simulink model "engine_64"  (R2022b)
settings: Solver=ode45  StartTime=0.0  StopTime=timeFinal  MaxStep=timeStepMax  RelTol=1e-3
settings Model: Creator=jun  LastModifiedBy=jun

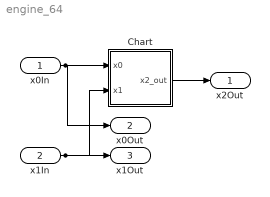
== system engine_64 ==
  x0In : Inport
  x1In : Inport  Port=2
  Chart : Stateflow chart  TreatAsAtomicUnit=on
  x2Out : Outport  SignalName=x2Out
  x0Out : Outport  Port=2  SignalName=x0Out
  x1Out : Outport  Port=3  SignalName=x1Out
  wires:
  x1In/1 -> x1Out/1, Chart/2(x1)
  Chart/1(x2_out) -> x2Out/1
  x0In/1 -> x0Out/1, Chart/1(x0)

== stateflow chart engine_64/Chart ==
  settings: updateMethod=CONTINUOUS  executeAtInitialization=1
  state loc1
    du:
    x2_dot = 172.1190893330591 * x0 + -18.178520839265644 * x1 + -0.5876147842465436 * x2 + 73.82076094915064 * 1;
    exit:
    x2_out = x2;
  state loc2
    du:
    x2_dot = 212.32859447747805 * x0 + -26.397573588389246 * x1 + -0.6081093746409181 * x2 + -30.45837836855404 * 1;
    exit:
    x2_out = x2;
  state loc3
    du:
    x2_dot = 344.54752773501156 * x0 + -35.88284070082604 * x1 + -0.9970388195562307 * x2 + -200.1049879468369 * 1;
    exit:
    x2_out = x2;
  state loc4
    du:
    x2_dot = 68.77841442397082 * x0 + -34.49189091176032 * x1 + 0.12328748344088325 * x2 + -1.3796756365879104 * 1;
    exit:
    x2_out = x2;
  state loc5
    du:
    x2_dot = 140.9675820907455 * x0 + -43.875858449678596 * x1 + -0.35477696051004415 * x2 + 521.9542303520906 * 1;
    exit:
    x2_out = x2;
  state loc6
    du:
    x2_dot = 302.8780197068835 * x0 + -44.80735860300237 * x1 + -0.9040556603935528 * x2 + 119.6620402089771 * 1;
    exit:
    x2_out = x2;
  state loc7
    du:
    x2_dot = 122.84651515781506 * x0 + -30.950644261836022 * x1 + -0.27788754543099614 * x2 + 165.80183448821774 * 1;
    exit:
    x2_out = x2;
  state loc8
    du:
    x2_dot = 167.10608158842408 * x0 + -108.5883262202008 * x1 + 0.009044623571327293 * x2 + 765.0984015639142 * 1;
    exit:
    x2_out = x2;
  state loc9
    du:
    x2_dot = 445.763959616979 * x0 + -48.47627467335269 * x1 + -2.0084227525216107 * x2 + 1229.5257992077045 * 1;
    exit:
    x2_out = x2;
  state loc10
    du:
    x2_dot = 498.3363297723553 * x0 + -608.1571396037069 * x1 + 2.2252382167093856 * x2 + -30.407856980192502 * 1;
    exit:
    x2_out = x2;
  state loc11
    du:
    x2_dot = 715.2746433139067 * x0 + -76.64137058300118 * x1 + -3.8995547737660843 * x2 + 4813.856810500421 * 1;
    exit:
    x2_out = x2;
  state loc12
    du:
    x2_dot = 101.74320415088494 * x0 + -1088.197236164022 * x1 + 10.09776041865507 * x2 + -54.40986180820271 * 1;
    exit:
    x2_out = x2;
  state loc13
    du:
    x2_dot = 0.9880803031927505 * x0 + 234.9676077852242 * x1 + -1.3449544898614079 * x2 + -2016.1925055525626 * 1;
    exit:
    x2_out = x2;
  state loc14
    du:
    x2_dot = 574.2410555812266 * x0 + -219.6862421234948 * x1 + -0.45181543339600694 * x2 + -8.78744968493992 * 1;
    exit:
    x2_out = x2;
  state loc15
    du:
    x2_dot = -113.62089642920859 * x0 + 1.4251893673222886 * x1 + 0.41547085892133473 * x2 + 0.07125946836611427 * 1;
    exit:
    x2_out = x2;
  state loc16
    du:
    x2_dot = -17.804841615106636 * x0 + -68.58762574035667 * x1 + 0.7167188324753084 * x2 + -3.4293812870178146 * 1;
    exit:
    x2_out = x2;
  state loc17
    du:
    x2_dot = 488.74438626957965 * x0 + 225.74711280684693 * x1 + -3.3008046366363715 * x2 + 11.287355640342154 * 1;
    exit:
    x2_out = x2;
  state loc18
    du:
    x2_dot = -468.38046258942035 * x0 + 2160.4248073159097 * x1 + -12.796021201925669 * x2 + 108.02124036578972 * 1;
    exit:
    x2_out = x2;
  state loc19
    du:
    x2_dot = 444.0255362071473 * x0 + -52.37346781168098 * x1 + -1.2930395931825203 * x2 + -108.66490645690529 * 1;
    exit:
    x2_out = x2;
  state loc20
    du:
    x2_dot = -869.7564517020274 * x0 + 109.0511700650369 * x1 + 2.8810707254181835 * x2 + -685.1892952940185 * 1;
    exit:
    x2_out = x2;
  state loc21
    du:
    x2_dot = 218.7833974995426 * x0 + -123.99564219310582 * x1 + -0.06817727388202854 * x2 + 761.9987134200146 * 1;
    exit:
    x2_out = x2;
  state loc22
    du:
    x2_dot = 788.4071927351927 * x0 + -119.82213911601772 * x1 + -2.006903759656254 * x2 + -5.991106955814446 * 1;
    exit:
    x2_out = x2;
  state loc23
    du:
    x2_dot = 423.7038947466738 * x0 + -43.16222518540387 * x1 + -1.3136762805154802 * x2 + -2.1581112592700946 * 1;
    exit:
    x2_out = x2;
  state loc24
    du:
    x2_dot = 994.6097170675433 * x0 + -203.68291006478168 * x1 + -2.1564190295835033 * x2 + -10.184145503239503 * 1;
    exit:
    x2_out = x2;
  state loc25
    du:
    x2_dot = 374.4538870917575 * x0 + -98.20167702486981 * x1 + -0.8107898899313994 * x2 + 419.8926588686644 * 1;
    exit:
    x2_out = x2;
  state loc26
    du:
    x2_dot = -244.70808961685935 * x0 + 19.943747525090956 * x1 + 0.7749081129909143 * x2 + 0.9971873762567732 * 1;
    exit:
    x2_out = x2;
  state loc27
    du:
    x2_dot = 411.98519906961934 * x0 + -620.8941581271833 * x1 + 2.744796134076182 * x2 + -31.04470790636005 * 1;
    exit:
    x2_out = x2;
  state loc28
    du:
    x2_dot = 808.0544999187772 * x0 + -453.71522052241687 * x1 + 0.16551686679935074 * x2 + -22.685761026118698 * 1;
    exit:
    x2_out = x2;
  state loc29
    du:
    x2_dot = 1233.9714475585872 * x0 + -154.78052698430878 * x1 + 1.7448402024567429 * x2 + -15821.406666081208 * 1;
    exit:
    x2_out = x2;
  state loc30
    du:
    x2_dot = 2676.133503156692 * x0 + -5868.971418919643 * x1 + 46.061341141875346 * x2 + -293.4485709459356 * 1;
    exit:
    x2_out = x2;
  state loc31
    du:
    x2_dot = 610.7207718994838 * x0 + -895.3235311192502 * x1 + 3.7777411657806397 * x2 + -44.76617655596021 * 1;
    exit:
    x2_out = x2;
  state loc32
    du:
    x2_dot = -3148.761851638217 * x0 + 10827.718842808368 * x1 + -93.44485779293609 * x2 + 541.3859421386076 * 1;
    exit:
    x2_out = x2;
  state loc33
    du:
    x2_dot = -12030.39472552258 * x0 + 25831.904809330747 * x1 + -205.25313427422952 * x2 + 1291.5952404673042 * 1;
    exit:
    x2_out = x2;
  state loc34
    du:
    x2_dot = 1263.8449377742227 * x0 + -2343.4654610634916 * x1 + 11.238228392457586 * x2 + -117.17327305316228 * 1;
    exit:
    x2_out = x2;
  state loc35
    du:
    x2_dot = 1182.9897670761286 * x0 + 2854.1817686159516 * x1 + -24.079857341380375 * x2 + 142.70908843089268 * 1;
    exit:
    x2_out = x2;
  state loc36
    du:
    x2_dot = 681.281153915759 * x0 + -678.712291850798 * x1 + 2.011639558995057 * x2 + -33.935614592536766 * 1;
    exit:
    x2_out = x2;
  state loc37
    du:
    x2_dot = 740.3742715734447 * x0 + 4.555906136101871 * x1 + -2.888094342106238 * x2 + 0.22779530681067664 * 1;
    exit:
    x2_out = x2;
  loc6 -> loc37 [order 20] : [ -1.0 * x0 + 0.0 * x1 + 0.013906389598449646 * x2 + -28.99226633725397 * 1 <= 0.000000 + 0]{x2 = 0.0 * x0 + 0.0 * x1 + 1.0 * x2 + 0.0; }
  loc31 -> loc2 [order 1] : [ 1.0 * x0 + 0.0 * x1 + -0.0004837518521937046 * x2 + -9.838665487841753 * 1 <= 0.000000 + 0]{x2 = 0.0 * x0 + 0.0 * x1 + 1.0 * x2 + 0.0; }
  loc30 -> loc1 [order 1] : [ 1.0 * x0 + 0.0 * x1 + 0.037800857937021634 * x2 + -86.5531921059513 * 1 <= 0.000000 + 0]{x2 = 0.0 * x0 + 0.0 * x1 + 1.0 * x2 + 0.0; }
  loc29 -> loc2 [order 1] : [ 1.0 * x0 + 0.0 * x1 + -0.003459682334038146 * x2 + -1.1898106761438398 * 1 <= 0.000000 + 0]{x2 = 0.0 * x0 + 0.0 * x1 + 1.0 * x2 + 0.0; }
  loc2 -> loc27 [order 16] : [ -1.0 * x0 + 0.0 * x1 + -0.04414154854203641 * x2 + 138.02065292561662 * 1 <= 0.000000 + 0]{x2 = 0.0 * x0 + 0.0 * x1 + 1.0 * x2 + 0.0; }
  loc29 -> loc5 [order 2] : [ 1.0 * x0 + 0.0 * x1 + -0.0006373591041330456 * x2 + -9.999681042268188 * 1 <= 0.000000 + 0]{x2 = 0.0 * x0 + 0.0 * x1 + 1.0 * x2 + 0.0; }
  loc27 -> loc5 [order 2] : [ 1.0 * x0 + 0.0 * x1 + -2.4418464604405856 * x2 + 7005.313200703071 * 1 <= 0.000000 + 0]{x2 = 0.0 * x0 + 0.0 * x1 + 1.0 * x2 + 0.0; }
  loc3 -> loc35 [order 15] : [ -1.0 * x0 + 0.0 * x1 + 0.013486455150813936 * x2 + -28.392022121626614 * 1 <= 0.000000 + 0]{x2 = 0.0 * x0 + 0.0 * x1 + 1.0 * x2 + 0.0; }
  loc1 -> loc32 [order 16] : [ -1.0 * x0 + 0.0 * x1 + 0.004088071137166638 * x2 + 0.2521195355914201 * 1 <= 0.000000 + 0]{x2 = 0.0 * x0 + 0.0 * x1 + 1.0 * x2 + 0.0; }
  loc25 -> loc6 [order 3] : [ -1.0 * x0 + 0.0 * x1 + 0.00966346036001345 * x2 + -17.678823102179155 * 1 <= 0.000000 + 0]{x2 = 0.0 * x0 + 0.0 * x1 + 1.0 * x2 + 0.0; }
  loc25 -> loc7 [order 4] : [ -1.0 * x0 + 0.0 * x1 + -0.0011937423705091499 * x2 + 15.265293647242267 * 1 <= 0.000000 + 0]{x2 = 0.0 * x0 + 0.0 * x1 + 1.0 * x2 + 0.0; }
  loc19 -> loc1 [order 1] : [ 1.0 * x0 + 0.0 * x1 + -4.5842158685289185e-05 * x2 + -8.34591726461707 * 1 <= 0.000000 + 0]{x2 = 0.0 * x0 + 0.0 * x1 + 1.0 * x2 + 0.0; }
  loc8 -> loc25 [order 13] : [ 1.0 * x0 + 0.0 * x1 + -0.008430233285089463 * x2 + 13.58360591452279 * 1 <= 0.000000 + 0]{x2 = 0.0 * x0 + 0.0 * x1 + 1.0 * x2 + 0.0; }
  loc28 -> loc11 [order 2] : [ -1.0 * x0 + 0.0 * x1 + 0.01341203766078607 * x2 + -28.164459590046405 * 1 <= 0.000000 + 0]{x2 = 0.0 * x0 + 0.0 * x1 + 1.0 * x2 + 0.0; }
  loc32 -> loc5 [order 1] : [ 1.0 * x0 + 0.0 * x1 + -0.02514010133359352 * x2 + 42.578630975660474 * 1 <= 0.000000 + 0]{x2 = 0.0 * x0 + 0.0 * x1 + 1.0 * x2 + 0.0; }
  loc20 -> loc5 [order 1] : [ -1.0 * x0 + 0.0 * x1 + 0.006990406418224249 * x2 + -5.009237016294506 * 1 <= 0.000000 + 0]{x2 = 0.0 * x0 + 0.0 * x1 + 1.0 * x2 + 0.0; }
  loc6 -> loc21 [order 14] : [ -1.0 * x0 + 0.0 * x1 + 0.002668645444580668 * x2 + 3.141070196132779 * 1 <= 0.000000 + 0]{x2 = 0.0 * x0 + 0.0 * x1 + 1.0 * x2 + 0.0; }
  loc6 -> loc31 [order 19] : [ -1.0 * x0 + 0.0 * x1 + 0.006683539436932168 * x2 + -8.706075096729139 * 1 <= 0.000000 + 0]{x2 = 0.0 * x0 + 0.0 * x1 + 1.0 * x2 + 0.0; }
  loc5 -> loc20 [order 15] : [ 1.0 * x0 + 0.0 * x1 + -0.0005830018611406415 * x2 + -7.805969915942764 * 1 <= 0.000000 + 0]{x2 = 0.0 * x0 + 0.0 * x1 + 1.0 * x2 + 0.0; }
  loc7 -> loc21 [order 8] : [ 1.0 * x0 + 0.0 * x1 + -0.011619069412716261 * x2 + 14.9354501584351 * 1 <= 0.000000 + 0]{x2 = 0.0 * x0 + 0.0 * x1 + 1.0 * x2 + 0.0; }
  loc5 -> loc18 [order 14] : [ 1.0 * x0 + 0.0 * x1 + -0.004338447137090646 * x2 + 1.1687838054601252 * 1 <= 0.000000 + 0]{x2 = 0.0 * x0 + 0.0 * x1 + 1.0 * x2 + 0.0; }
  loc1 -> loc14 [order 11] : [ -1.0 * x0 + 0.0 * x1 + 0.011364322618163452 * x2 + -21.491953472474837 * 1 <= 0.000000 + 0]{x2 = 0.0 * x0 + 0.0 * x1 + 1.0 * x2 + 0.0; }
  loc2 -> loc15 [order 11] : [ 1.0 * x0 + 0.0 * x1 + -0.005246642341844816 * x2 + 4.512806263509677 * 1 <= 0.000000 + 0]{x2 = 0.0 * x0 + 0.0 * x1 + 1.0 * x2 + 0.0; }
  loc2 -> loc23 [order 15] : [ -1.0 * x0 + 0.0 * x1 + -0.0066847022325267 * x2 + 31.03761365685755 * 1 <= 0.000000 + 0]{x2 = 0.0 * x0 + 0.0 * x1 + 1.0 * x2 + 0.0; }
  loc21 -> loc1 [order 1] : [ 1.0 * x0 + 0.0 * x1 + -0.03785322377042109 * x2 + 68.62399585559116 * 1 <= 0.000000 + 0]{x2 = 0.0 * x0 + 0.0 * x1 + 1.0 * x2 + 0.0; }
  loc17 -> loc6 [order 2] : [ 1.0 * x0 + 0.0 * x1 + 0.007876696914691554 * x2 + -35.52805351984629 * 1 <= 0.000000 + 0]{x2 = 0.0 * x0 + 0.0 * x1 + 1.0 * x2 + 0.0; }
  loc19 -> loc2 [order 2] : [ -1.0 * x0 + 2.1501424257403646e-14 * x1 + -0.49815175716791427 * x2 + 1497.204463041921 * 1 <= 0.000000 + 0]{x2 = 0.0 * x0 + 0.0 * x1 + 1.0 * x2 + 0.0; }
  loc25 -> loc8 [order 5] : [ 1.0 * x0 + 0.0 * x1 + -0.01386269505556377 * x2 + 19.586861582100134 * 1 <= 0.000000 + 0]{x2 = 0.0 * x0 + 0.0 * x1 + 1.0 * x2 + 0.0; }
  loc3 -> loc13 [order 10] : [ -1.0 * x0 + 0.0 * x1 + 0.00850238412940428 * x2 + -8.6891486981035 * 1 <= 0.000000 + 0]{x2 = 0.0 * x0 + 0.0 * x1 + 1.0 * x2 + 0.0; }
  loc16 -> loc6 [order 2] : [ -1.0 * x0 + 0.0 * x1 + 0.0010295685996749922 * x2 + 6.426480142622885 * 1 <= 0.000000 + 0]{x2 = 0.0 * x0 + 0.0 * x1 + 1.0 * x2 + 0.0; }
  loc9 -> loc1 [order 1] : [ 1.0 * x0 + 0.0 * x1 + 0.008495833391664445 * x2 + -25.608980012374634 * 1 <= 0.000000 + 0]{x2 = 0.0 * x0 + 0.0 * x1 + 1.0 * x2 + 0.0; }
  loc2 -> loc10 [order 10] : [ -1.0 * x0 + 0.0 * x1 + 0.013652563074296183 * x2 + -29.304627262579817 * 1 <= 0.000000 + 0]{x2 = 0.0 * x0 + 0.0 * x1 + 1.0 * x2 + 0.0; }
  loc13 -> loc21 [order 10] : [ -1.0 * x0 + 0.0 * x1 + 0.23556519772450607 * x2 + -669.100757040598 * 1 <= 0.000000 + 0]{x2 = 0.0 * x0 + 0.0 * x1 + 1.0 * x2 + 0.0; }
  loc8 -> loc21 [order 12] : [ 0.0 * x0 + 0.0 * x1 + -3.7019148417951926 * x2 + 7502.2921311782975 * 1 <= 0.000000 + 0]{x2 = 0.0 * x0 + 0.0 * x1 + 1.0 * x2 + 0.0; }
  loc6 -> loc19 [order 13] : [ -1.0 * x0 + 0.0 * x1 + 0.07262992925696107 * x2 + -136.64188709123505 * 1 <= 0.000000 + 0]{x2 = 0.0 * x0 + 0.0 * x1 + 1.0 * x2 + 0.0; }
  loc13 -> loc5 [order 4] : [ 1.0 * x0 + 0.0 * x1 + 0.0166038325905201 * x2 + -42.09105224715482 * 1 <= 0.000000 + 0]{x2 = 0.0 * x0 + 0.0 * x1 + 1.0 * x2 + 0.0; }
  loc13 -> loc6 [order 5] : [ -1.0 * x0 + 0.0 * x1 + 0.004000795211689418 * x2 + 0.3168817954571548 * 1 <= 0.000000 + 0]{x2 = 0.0 * x0 + 0.0 * x1 + 1.0 * x2 + 0.0; }
  loc1 -> loc13 [order 10] : [ -1.0 * x0 + 0.0 * x1 + 0.010412265577585919 * x2 + -15.559847318348758 * 1 <= 0.000000 + 0]{x2 = 0.0 * x0 + 0.0 * x1 + 1.0 * x2 + 0.0; }
  loc8 -> loc1 [order 1] : [ 1.0 * x0 + 0.0 * x1 + -0.0011841946054482308 * x2 + -6.817120131792731 * 1 <= 0.000000 + 0]{x2 = 0.0 * x0 + 0.0 * x1 + 1.0 * x2 + 0.0; }
  loc7 -> loc1 [order 1] : [ -1.0 * x0 + 0.0 * x1 + -0.000396194716564098 * x2 + 10.813484261025486 * 1 <= 0.000000 + 0]{x2 = 0.0 * x0 + 0.0 * x1 + 1.0 * x2 + 0.0; }
  loc7 -> loc2 [order 2] : [ 1.0 * x0 + 1.9355245087005833e-14 * x1 + -0.5842959775119011 * x2 + 1696.0577007802651 * 1 <= 0.000000 + 0]{x2 = 0.0 * x0 + 0.0 * x1 + 1.0 * x2 + 0.0; }
  loc10 -> loc2 [order 1] : [ -1.0 * x0 + 0.0 * x1 + -0.008129878521809913 * x2 + 35.3429710977038 * 1 <= 0.000000 + 0]{x2 = 0.0 * x0 + 0.0 * x1 + 1.0 * x2 + 0.0; }
  loc1 -> loc6 [order 5] : [ -1.0 * x0 + 1.920474508744948e-15 * x1 + 0.002396822510459467 * x2 + 3.886275756636265 * 1 <= 0.000000 + 0]{x2 = 0.0 * x0 + 0.0 * x1 + 1.0 * x2 + 0.0; }
  loc2 -> loc9 [order 9] : [ 1.0 * x0 + 0.0 * x1 + -0.0004847832930982423 * x2 + -8.002702057926387 * 1 <= 0.000000 + 0]{x2 = 0.0 * x0 + 0.0 * x1 + 1.0 * x2 + 0.0; }
  loc6 -> loc2 [order 2] : [ -1.0 * x0 + -2.2612069380927382e-14 * x1 + 0.0008976844746347977 * x2 + 7.987968808200821 * 1 <= 0.000000 + 0]{x2 = 0.0 * x0 + 0.0 * x1 + 1.0 * x2 + 0.0; }
  loc5 -> loc9 [order 9] : [ 1.0 * x0 + 0.0 * x1 + -0.02627481784478791 * x2 + 44.3802704365903 * 1 <= 0.000000 + 0]{x2 = 0.0 * x0 + 0.0 * x1 + 1.0 * x2 + 0.0; }
  loc3 -> loc9 [order 9] : [ 1.0 * x0 + 0.0 * x1 + 0.02989985141165207 * x2 + -68.67750395221753 * 1 <= 0.000000 + 0]{x2 = 0.0 * x0 + 0.0 * x1 + 1.0 * x2 + 0.0; }
  loc8 -> loc2 [order 2] : [ 1.0 * x0 + 0.0 * x1 + -0.004360712734463186 * x2 + 0.924986077398196 * 1 <= 0.000000 + 0]{x2 = 0.0 * x0 + 0.0 * x1 + 1.0 * x2 + 0.0; }
  loc5 -> loc8 [order 8] : [ -1.0 * x0 + 0.0 * x1 + -0.3165002257184714 * x2 + 802.3004669529307 * 1 <= 0.000000 + 0]{x2 = 0.0 * x0 + 0.0 * x1 + 1.0 * x2 + 0.0; }
  loc16 -> loc13 [order 3] : [ -1.0 * x0 + 0.0 * x1 + 0.003592581833683608 * x2 + 0.8675894511976858 * 1 <= 0.000000 + 0]{x2 = 0.0 * x0 + 0.0 * x1 + 1.0 * x2 + 0.0; }
  loc6 -> loc9 [order 8] : [ 1.0 * x0 + 0.0 * x1 + 0.012514221631630334 * x2 + -33.66438324655323 * 1 <= 0.000000 + 0]{x2 = 0.0 * x0 + 0.0 * x1 + 1.0 * x2 + 0.0; }
  loc1 -> loc5 [order 4] : [ -1.0 * x0 + -2.6266718131235672e-14 * x1 + 0.0008845513854542847 * x2 + 7.954499085333239 * 1 <= 0.000000 + 0]{x2 = 0.0 * x0 + 0.0 * x1 + 1.0 * x2 + 0.0; }
  loc5 -> loc2 [order 2] : [ 1.0 * x0 + 5.0921810950735284e-14 * x1 + -0.02049676115225059 * x2 + 41.34643404703749 * 1 <= 0.000000 + 0]{x2 = 0.0 * x0 + 0.0 * x1 + 1.0 * x2 + 0.0; }
  loc2 -> loc5 [order 5] : [ -1.0 * x0 + -6.107671307757277e-14 * x1 + -0.1353375334038646 * x2 + 411.09517067157344 * 1 <= 0.000000 + 0]{x2 = 0.0 * x0 + 0.0 * x1 + 1.0 * x2 + 0.0; }
  loc7 -> loc3 [order 3] : [ 1.0 * x0 + 0.0 * x1 + -0.0010294929919228354 * x2 + -7.2614381063231885 * 1 <= 0.000000 + 0]{x2 = 0.0 * x0 + 0.0 * x1 + 1.0 * x2 + 0.0; }
  loc2 -> loc4 [order 4] : [ 1.0 * x0 + 0.0 * x1 + -0.00016505883538827908 * x2 + -8.64187436094922 * 1 <= 0.000000 + 0]{x2 = 0.0 * x0 + 0.0 * x1 + 1.0 * x2 + 0.0; }
  loc5 -> loc3 [order 3] : [ 1.0 * x0 + 0.0 * x1 + -0.0008682788409220731 * x2 + -7.647835038707683 * 1 <= 0.000000 + 0]{x2 = 0.0 * x0 + 0.0 * x1 + 1.0 * x2 + 0.0; }
  loc6 -> loc3 [order 3] : [ 1.0 * x0 + 0.0 * x1 + 0.019351697137556877 * x2 + -58.86799090745678 * 1 <= 0.000000 + 0]{x2 = 0.0 * x0 + 0.0 * x1 + 1.0 * x2 + 0.0; }
  loc6 -> loc8 [order 7] : [ -1.0 * x0 + 0.0 * x1 + 0.01900167156417144 * x2 + -29.88892120409554 * 1 <= 0.000000 + 0]{x2 = 0.0 * x0 + 0.0 * x1 + 1.0 * x2 + 0.0; }
  loc7 -> loc8 [order 7] : [ 1.0 * x0 + 0.0 * x1 + -0.04280097395098223 * x2 + 93.25578195856991 * 1 <= 0.000000 + 0]{x2 = 0.0 * x0 + 0.0 * x1 + 1.0 * x2 + 0.0; }
  loc18 -> loc19 [order 1] : [ -1.0 * x0 + 0.0 * x1 + -0.0007374404508494473 * x2 + 13.516688409477354 * 1 <= 0.000000 + 0]{x2 = 0.0 * x0 + 0.0 * x1 + 1.0 * x2 + 0.0; }
  loc3 -> loc4 [order 4] : [ 1.0 * x0 + 0.0 * x1 + 0.001053045477463381 * x2 + -11.078191168027793 * 1 <= 0.000000 + 0]{x2 = 0.0 * x0 + 0.0 * x1 + 1.0 * x2 + 0.0; }
  loc5 -> loc4 [order 4] : [ 1.0 * x0 + 0.0 * x1 + -0.0002327516748476991 * x2 + -8.506449954332243 * 1 <= 0.000000 + 0]{x2 = 0.0 * x0 + 0.0 * x1 + 1.0 * x2 + 0.0; }
  loc2 -> loc3 [order 3] : [ 1.0 * x0 + 2.587408275651915e-14 * x1 + -0.00033074273625259185 * x2 + -9.139048550165036 * 1 <= 0.000000 + 0]{x2 = 0.0 * x0 + 0.0 * x1 + 1.0 * x2 + 0.0; }
  loc9 -> loc8 [order 6] : [ 1.0 * x0 + 0.0 * x1 + 0.0002770668648333768 * x2 + -8.995542602209866 * 1 <= 0.000000 + 0]{x2 = 0.0 * x0 + 0.0 * x1 + 1.0 * x2 + 0.0; }
  (junction 38) -> loc1 : [-1.0 * x0 + 9.775494234578627e-15 * x1 + 0.0121850121227071 * x2 + -21.54718632368986 * 1 <= 0.000000 + 0]{x2 = 0.0 * x0 + 0.0 * x1 + 1.0 * x2 + 0.0; }
  (default) -> loc1 : {x2 = a2; }
  (junction 77) -> loc2 : {x2 = x2; }
  (junction 60) -> loc2 : [-1.0 * x0 + 1.80572554083749e-15 * x1 + -0.0897209572126218 * x2 + 275.1294182888892 * 1 <= 0.000000 + 0]{x2 = 0.0 * x0 + 0.0 * x1 + 1.0 * x2 + 0.0; }
  (junction 97) -> loc3 : {x2 = x2; }
  (junction 82) -> loc3 : [1.0 * x0 + 0.0 * x1 + 0.005128621719638715 * x2 + -22.854840694945942 * 1 <= 0.000000 + 0]{x2 = 0.0 * x0 + 0.0 * x1 + 1.0 * x2 + 0.0; }
  (junction 101) -> loc4 : {x2 = x2; }
  (junction 125) -> loc5 : {x2 = x2; }
  (junction 108) -> loc5 : [1.0 * x0 + -8.853049182917268e-14 * x1 + -0.05600468311549547 * x2 + 125.14797413040408 * 1 <= 0.000000 + 0]{x2 = 0.0 * x0 + 0.0 * x1 + 1.0 * x2 + 0.0; }
  (junction 150) -> loc6 : {x2 = x2; }
  (junction 132) -> loc6 : [-1.0 * x0 + 8.119871136734383e-15 * x1 + 0.0043214885731190705 * x2 + -0.7481009740519966 * 1 <= 0.000000 + 0]{x2 = 0.0 * x0 + 0.0 * x1 + 1.0 * x2 + 0.0; }
  (junction 163) -> loc7 : {x2 = x2; }
  (junction 158) -> loc7 : [-1.0 * x0 + 2.3628053529496597e-15 * x1 + -0.0012646308978708435 * x2 + 14.00654036505749 * 1 <= 0.000000 + 0]{x2 = 0.0 * x0 + 0.0 * x1 + 1.0 * x2 + 0.0; }
  (junction 184) -> loc8 : {x2 = x2; }
  (junction 172) -> loc8 : [1.0 * x0 + 0.0 * x1 + -0.15658104490158298 * x2 + 373.13046083466145 * 1 <= 0.000000 + 0]{x2 = 0.0 * x0 + 0.0 * x1 + 1.0 * x2 + 0.0; }
  (junction 193) -> loc9 : {x2 = x2; }
  (junction 197) -> loc10 : {x2 = x2; }
  (junction 203) -> loc11 : {x2 = x2; }
  (junction 208) -> loc12 : {x2 = x2; }
  (junction 223) -> loc13 : {x2 = x2; }
  (junction 219) -> loc13 : [-1.0 * x0 + 0.0 * x1 + 0.003075190697417944 * x2 + 2.1890451934694903 * 1 <= 0.000000 + 0]{x2 = 0.0 * x0 + 0.0 * x1 + 1.0 * x2 + 0.0; }
  (junction 228) -> loc14 : {x2 = x2; }
  (junction 233) -> loc15 : {x2 = x2; }
  (junction 239) -> loc16 : {x2 = x2; }
  (junction 245) -> loc17 : {x2 = x2; }
  (junction 249) -> loc18 : {x2 = x2; }
  (junction 256) -> loc19 : {x2 = x2; }
  (junction 261) -> loc20 : {x2 = x2; }
  (junction 268) -> loc21 : {x2 = x2; }
  (junction 273) -> loc22 : {x2 = x2; }
  (junction 279) -> loc23 : {x2 = x2; }
  (junction 284) -> loc24 : {x2 = x2; }
  (junction 292) -> loc25 : {x2 = x2; }
  (junction 297) -> loc26 : {x2 = x2; }
  (junction 302) -> loc27 : {x2 = x2; }
  (junction 308) -> loc28 : {x2 = x2; }
  (junction 313) -> loc29 : {x2 = x2; }
  (junction 317) -> loc30 : {x2 = x2; }
  (junction 321) -> loc31 : {x2 = x2; }
  (junction 325) -> loc32 : {x2 = x2; }
  (junction 329) -> loc33 : {x2 = x2; }
  (junction 333) -> loc34 : {x2 = x2; }
  (junction 337) -> loc35 : {x2 = x2; }
  (junction 341) -> loc36 : {x2 = x2; }
  (junction 345) -> loc37 : {x2 = x2; }
  loc1 -> (junction 56) [order 17]
  (junction 56) -> loc1 : {x2 = x2; }
  loc1 -> (junction 38) [order 1]
  loc2 -> (junction 77) [order 17]
  loc2 -> (junction 60) [order 2]
  loc3 -> (junction 97) [order 16]
  loc3 -> (junction 82) [order 3]
  loc4 -> (junction 101) [order 2]
  loc5 -> (junction 125) [order 20]
  loc5 -> (junction 108) [order 5]
  loc6 -> (junction 150) [order 21]
  loc6 -> (junction 132) [order 5]
  loc7 -> (junction 163) [order 9]
  loc7 -> (junction 158) [order 6]
  loc8 -> (junction 184) [order 17]
  loc8 -> (junction 172) [order 7]
  loc9 -> (junction 193) [order 7]
  loc10 -> (junction 197) [order 2]
  loc11 -> (junction 203) [order 4]
  loc12 -> (junction 208) [order 3]
  loc13 -> (junction 223) [order 11]
  loc13 -> (junction 219) [order 9]
  loc14 -> (junction 228) [order 3]
  loc15 -> (junction 233) [order 3]
  loc16 -> (junction 239) [order 4]
  loc17 -> (junction 245) [order 4]
  loc18 -> (junction 249) [order 2]
  loc19 -> (junction 256) [order 5]
  loc20 -> (junction 261) [order 3]
  loc21 -> (junction 268) [order 5]
  loc22 -> (junction 273) [order 3]
  loc23 -> (junction 279) [order 4]
  loc24 -> (junction 284) [order 3]
  loc25 -> (junction 292) [order 6]
  loc26 -> (junction 297) [order 3]
  loc27 -> (junction 302) [order 3]
  loc28 -> (junction 308) [order 4]
  loc29 -> (junction 313) [order 3]
  loc30 -> (junction 317) [order 2]
  loc31 -> (junction 321) [order 2]
  loc32 -> (junction 325) [order 2]
  loc33 -> (junction 329) [order 2]
  loc34 -> (junction 333) [order 2]
  loc35 -> (junction 337) [order 2]
  loc36 -> (junction 341) [order 2]
  loc37 -> (junction 345) [order 2]
  loc6 -> loc11 [order 9] : [ -1.0 * x0 + 0.0 * x1 + 0.003061995106964173 * x2 + 2.727600433090311 * 1 <= 0.000000 + 0]{x2 = 0.0 * x0 + 0.0 * x1 + 1.0 * x2 + 0.0; }
  loc6 -> loc24 [order 15] : [ 1.0 * x0 + 0.0 * x1 + 0.0003851795086086663 * x2 + -9.224248852383578 * 1 <= 0.000000 + 0]{x2 = 0.0 * x0 + 0.0 * x1 + 1.0 * x2 + 0.0; }
  loc17 -> loc36 [order 3] : [ -1.0 * x0 + 0.0 * x1 + 0.0078073515693894355 * x2 + -12.275851653089429 * 1 <= 0.000000 + 0]{x2 = 0.0 * x0 + 0.0 * x1 + 1.0 * x2 + 0.0; }
  loc8 -> loc13 [order 8] : [ 1.0 * x0 + 0.0 * x1 + -0.41473185044808303 * x2 + 833.6030054148777 * 1 <= 0.000000 + 0]{x2 = 0.0 * x0 + 0.0 * x1 + 1.0 * x2 + 0.0; }
  loc8 -> loc28 [order 14] : [ 1.0 * x0 + 0.0 * x1 + -0.0008137390729368074 * x2 + -9.884470033609494 * 1 <= 0.000000 + 0]{x2 = 0.0 * x0 + 0.0 * x1 + 1.0 * x2 + 0.0; }
  loc28 -> loc29 [order 3] : [ -1.0 * x0 + 0.0 * x1 + 0.01198396513255497 * x2 + -23.96741959343518 * 1 <= 0.000000 + 0]{x2 = 0.0 * x0 + 0.0 * x1 + 1.0 * x2 + 0.0; }
  loc28 -> loc5 [order 1] : [ -1.0 * x0 + 0.0 * x1 + 0.014221919409240433 * x2 + -30.244302553187396 * 1 <= 0.000000 + 0]{x2 = 0.0 * x0 + 0.0 * x1 + 1.0 * x2 + 0.0; }
  loc8 -> loc7 [order 6] : [ 1.0 * x0 + 0.0 * x1 + -0.0005897625708588623 * x2 + -9.820014728923372 * 1 <= 0.000000 + 0]{x2 = 0.0 * x0 + 0.0 * x1 + 1.0 * x2 + 0.0; }
  loc1 -> loc7 [order 6] : [ -1.0 * x0 + 0.0 * x1 + 0.0006725296527658178 * x2 + 8.44586008456916 * 1 <= 0.000000 + 0]{x2 = 0.0 * x0 + 0.0 * x1 + 1.0 * x2 + 0.0; }
  loc1 -> loc16 [order 12] : [ -1.0 * x0 + 0.0 * x1 + 0.006938432653440454 * x2 + -5.844851815434497 * 1 <= 0.000000 + 0]{x2 = 0.0 * x0 + 0.0 * x1 + 1.0 * x2 + 0.0; }
  loc17 -> loc1 [order 1] : [ -1.0 * x0 + 0.0 * x1 + 0.009958076561476438 * x2 + -18.52621545079124 * 1 <= 0.000000 + 0]{x2 = 0.0 * x0 + 0.0 * x1 + 1.0 * x2 + 0.0; }
  loc26 -> loc13 [order 2] : [ -1.0 * x0 + 0.0 * x1 + 0.005272701492981822 * x2 + -2.24677477710992 * 1 <= 0.000000 + 0]{x2 = 0.0 * x0 + 0.0 * x1 + 1.0 * x2 + 0.0; }
  loc6 -> loc1 [order 1] : [ -1.0 * x0 + 5.2775269187444e-15 * x1 + 0.0018543047641648885 * x2 + 5.461340165715162 * 1 <= 0.000000 + 0]{x2 = 0.0 * x0 + 0.0 * x1 + 1.0 * x2 + 0.0; }
  loc3 -> loc5 [order 5] : [ -1.0 * x0 + 5.419359270896986e-16 * x1 + 6.766680895445332e-06 * x2 + 9.776387147649764 * 1 <= 0.000000 + 0]{x2 = 0.0 * x0 + 0.0 * x1 + 1.0 * x2 + 0.0; }
  loc3 -> loc24 [order 11] : [ -1.0 * x0 + 0.0 * x1 + 0.00020032908282740537 * x2 + 8.055033640322778 * 1 <= 0.000000 + 0]{x2 = 0.0 * x0 + 0.0 * x1 + 1.0 * x2 + 0.0; }
  loc15 -> loc6 [order 2] : [ -1.0 * x0 + 0.0 * x1 + 0.01247769896472895 * x2 + -24.822269825283854 * 1 <= 0.000000 + 0]{x2 = 0.0 * x0 + 0.0 * x1 + 1.0 * x2 + 0.0; }
  loc13 -> loc3 [order 3] : [ 1.0 * x0 + 0.0 * x1 + 0.0004328989487972267 * x2 + -9.385572117121479 * 1 <= 0.000000 + 0]{x2 = 0.0 * x0 + 0.0 * x1 + 1.0 * x2 + 0.0; }
  loc5 -> loc12 [order 10] : [ 1.0 * x0 + 0.0 * x1 + -0.15172077374063186 * x2 + 305.2791759295456 * 1 <= 0.000000 + 0]{x2 = 0.0 * x0 + 0.0 * x1 + 1.0 * x2 + 0.0; }
  loc5 -> loc22 [order 16] : [ 1.0 * x0 + 0.0 * x1 + -0.0007949504326678048 * x2 + -7.575308489923387 * 1 <= 0.000000 + 0]{x2 = 0.0 * x0 + 0.0 * x1 + 1.0 * x2 + 0.0; }
  loc9 -> loc7 [order 5] : [ 1.0 * x0 + 0.0 * x1 + 0.0011003152683534661 * x2 + -10.652779963478437 * 1 <= 0.000000 + 0]{x2 = 0.0 * x0 + 0.0 * x1 + 1.0 * x2 + 0.0; }
  loc9 -> loc3 [order 2] : [ 1.0 * x0 + 0.0 * x1 + 0.000505959707536987 * x2 + -9.50844114152303 * 1 <= 0.000000 + 0]{x2 = 0.0 * x0 + 0.0 * x1 + 1.0 * x2 + 0.0; }
  loc27 -> loc2 [order 1] : [ 1.0 * x0 + 0.0 * x1 + -0.003973753558748778 * x2 + 0.22232396459730006 * 1 <= 0.000000 + 0]{x2 = 0.0 * x0 + 0.0 * x1 + 1.0 * x2 + 0.0; }
  loc20 -> loc6 [order 2] : [ -1.0 * x0 + 0.0 * x1 + 0.003266853868709181 * x2 + 1.8536354335135146 * 1 <= 0.000000 + 0]{x2 = 0.0 * x0 + 0.0 * x1 + 1.0 * x2 + 0.0; }
  loc16 -> loc1 [order 1] : [ -1.0 * x0 + 0.0 * x1 + 0.07875374856763548 * x2 + -155.01450193772223 * 1 <= 0.000000 + 0]{x2 = 0.0 * x0 + 0.0 * x1 + 1.0 * x2 + 0.0; }
  loc2 -> loc6 [order 6] : [ -1.0 * x0 + 0.0 * x1 + -0.0007583640662728963 * x2 + 11.824030994291618 * 1 <= 0.000000 + 0]{x2 = 0.0 * x0 + 0.0 * x1 + 1.0 * x2 + 0.0; }
  loc2 -> loc17 [order 12] : [ 1.0 * x0 + 0.0 * x1 + -0.005947958362593438 * x2 + 6.6352236195673795 * 1 <= 0.000000 + 0]{x2 = 0.0 * x0 + 0.0 * x1 + 1.0 * x2 + 0.0; }
  loc11 -> loc2 [order 1] : [ -1.0 * x0 + 1.038173439278966e-15 * x1 + -0.01497800762556828 * x2 + 55.39052847424546 * 1 <= 0.000000 + 0]{x2 = 0.0 * x0 + 0.0 * x1 + 1.0 * x2 + 0.0; }
  loc5 -> loc1 [order 1] : [ 1.0 * x0 + 0.0 * x1 + -0.0037659877969931253 * x2 + -3.4088490147256745 * 1 <= 0.000000 + 0]{x2 = 0.0 * x0 + 0.0 * x1 + 1.0 * x2 + 0.0; }
  loc25 -> loc5 [order 2] : [ 1.0 * x0 + 0.0 * x1 + -0.0019058969268201038 * x2 + -6.262145480107898 * 1 <= 0.000000 + 0]{x2 = 0.0 * x0 + 0.0 * x1 + 1.0 * x2 + 0.0; }
  loc22 -> loc1 [order 1] : [ 1.0 * x0 + 0.0 * x1 + 0.0023917990139339113 * x2 + -13.277508973591443 * 1 <= 0.000000 + 0]{x2 = 0.0 * x0 + 0.0 * x1 + 1.0 * x2 + 0.0; }
  loc14 -> loc7 [order 2] : [ -1.0 * x0 + 0.0 * x1 + -0.00010976259879964654 * x2 + 12.170762386927034 * 1 <= 0.000000 + 0]{x2 = 0.0 * x0 + 0.0 * x1 + 1.0 * x2 + 0.0; }
  loc33 -> loc1 [order 1] : [ 1.0 * x0 + 0.0 * x1 + -0.03948316276394554 * x2 + 71.57094894860053 * 1 <= 0.000000 + 0]{x2 = 0.0 * x0 + 0.0 * x1 + 1.0 * x2 + 0.0; }
  loc5 -> loc31 [order 19] : [ -1.0 * x0 + 0.0 * x1 + 0.012647303790680344 * x2 + -26.017398529515656 * 1 <= 0.000000 + 0]{x2 = 0.0 * x0 + 0.0 * x1 + 1.0 * x2 + 0.0; }
  loc5 -> loc17 [order 13] : [ 1.0 * x0 + 0.0 * x1 + -0.0342194785085502 * x2 + 89.03909031132191 * 1 <= 0.000000 + 0]{x2 = 0.0 * x0 + 0.0 * x1 + 1.0 * x2 + 0.0; }
  loc5 -> loc7 [order 7] : [ 1.0 * x0 + 1.0497042541398529e-14 * x1 + -0.06454385484297653 * x2 + 179.085359195857 * 1 <= 0.000000 + 0]{x2 = 0.0 * x0 + 0.0 * x1 + 1.0 * x2 + 0.0; }
  loc13 -> loc7 [order 6] : [ -1.0 * x0 + 0.0 * x1 + 0.009965047282821127 * x2 + -11.640134730979971 * 1 <= 0.000000 + 0]{x2 = 0.0 * x0 + 0.0 * x1 + 1.0 * x2 + 0.0; }
  loc3 -> loc2 [order 2] : [ -1.0 * x0 + 4.5418127346750425e-14 * x1 + 0.00013355281121914993 * x2 + 9.757482433422817 * 1 <= 0.000000 + 0]{x2 = 0.0 * x0 + 0.0 * x1 + 1.0 * x2 + 0.0; }
  loc23 -> loc7 [order 3] : [ -1.0 * x0 + 0.0 * x1 + -0.0014075887513039208 * x2 + 15.529621022516077 * 1 <= 0.000000 + 0]{x2 = 0.0 * x0 + 0.0 * x1 + 1.0 * x2 + 0.0; }
  loc6 -> loc13 [order 10] : [ -1.0 * x0 + 0.0 * x1 + 0.0010309254441385057 * x2 + 6.403818135254402 * 1 <= 0.000000 + 0]{x2 = 0.0 * x0 + 0.0 * x1 + 1.0 * x2 + 0.0; }
  loc6 -> loc25 [order 16] : [ -1.0 * x0 + 0.0 * x1 + 0.0025629308305147795 * x2 + 4.235969786679616 * 1 <= 0.000000 + 0]{x2 = 0.0 * x0 + 0.0 * x1 + 1.0 * x2 + 0.0; }
  loc3 -> loc28 [order 14] : [ 1.0 * x0 + 0.0 * x1 + 0.007080093946932203 * x2 + -22.66942981864244 * 1 <= 0.000000 + 0]{x2 = 0.0 * x0 + 0.0 * x1 + 1.0 * x2 + 0.0; }
  loc3 -> loc8 [order 8] : [ 1.0 * x0 + 0.0 * x1 + 0.0017809738099518358 * x2 + -12.045092740766119 * 1 <= 0.000000 + 0]{x2 = 0.0 * x0 + 0.0 * x1 + 1.0 * x2 + 0.0; }
  loc21 -> loc8 [order 4] : [ 1.0 * x0 + 0.0 * x1 + -0.03895273970692649 * x2 + 70.55674837716509 * 1 <= 0.000000 + 0]{x2 = 0.0 * x0 + 0.0 * x1 + 1.0 * x2 + 0.0; }
  loc6 -> loc5 [order 4] : [ -1.0 * x0 + 5.407699530279431e-15 * x1 + 0.0007595768107165269 * x2 + 8.305979837030566 * 1 <= 0.000000 + 0]{x2 = 0.0 * x0 + 0.0 * x1 + 1.0 * x2 + 0.0; }
  loc8 -> loc15 [order 9] : [ 1.0 * x0 + 0.0 * x1 + -0.005011551395085967 * x2 + 3.2976229610623493 * 1 <= 0.000000 + 0]{x2 = 0.0 * x0 + 0.0 * x1 + 1.0 * x2 + 0.0; }
  loc8 -> loc33 [order 15] : [ 0.0 * x0 + 0.0 * x1 + -1.3390169825018456 * x2 + 2708.0949137445386 * 1 <= 0.000000 + 0]{x2 = 0.0 * x0 + 0.0 * x1 + 1.0 * x2 + 0.0; }
  loc1 -> loc26 [order 15] : [ 1.0 * x0 + 0.0 * x1 + 0.05263480188426551 * x2 + -117.10800060444946 * 1 <= 0.000000 + 0]{x2 = 0.0 * x0 + 0.0 * x1 + 1.0 * x2 + 0.0; }
  loc1 -> loc11 [order 9] : [ -1.0 * x0 + 0.0 * x1 + 0.011248132622429406 * x2 + -21.471717498578933 * 1 <= 0.000000 + 0]{x2 = 0.0 * x0 + 0.0 * x1 + 1.0 * x2 + 0.0; }
  loc1 -> loc3 [order 3] : [ 1.0 * x0 + 0.0 * x1 + 0.006381097929252417 * x2 + -21.377894493662033 * 1 <= 0.000000 + 0]{x2 = 0.0 * x0 + 0.0 * x1 + 1.0 * x2 + 0.0; }
  loc8 -> loc3 [order 3] : [ 1.0 * x0 + 0.0 * x1 + -0.00037710862038303945 * x2 + -7.737294429659588 * 1 <= 0.000000 + 0]{x2 = 0.0 * x0 + 0.0 * x1 + 1.0 * x2 + 0.0; }
  loc8 -> loc6 [order 5] : [ 1.0 * x0 + 0.0 * x1 + -0.006098390267404411 * x2 + 6.84350098886884 * 1 <= 0.000000 + 0]{x2 = 0.0 * x0 + 0.0 * x1 + 1.0 * x2 + 0.0; }
  loc1 -> loc8 [order 7] : [ -1.0 * x0 + 0.0 * x1 + 0.005134281914280692 * x2 + -1.8329947097038581 * 1 <= 0.000000 + 0]{x2 = 0.0 * x0 + 0.0 * x1 + 1.0 * x2 + 0.0; }
  loc1 -> loc21 [order 13] : [ 1.0 * x0 + 0.0 * x1 + 0.0053863416494962565 * x2 + -19.553885217411892 * 1 <= 0.000000 + 0]{x2 = 0.0 * x0 + 0.0 * x1 + 1.0 * x2 + 0.0; }
  loc3 -> loc6 [order 6] : [ -1.0 * x0 + 0.0 * x1 + 0.00454453084177528 * x2 + -1.5233219217089815 * 1 <= 0.000000 + 0]{x2 = 0.0 * x0 + 0.0 * x1 + 1.0 * x2 + 0.0; }
  loc3 -> loc25 [order 12] : [ -1.0 * x0 + 0.0 * x1 + 0.009463222472532354 * x2 + -15.809204975439513 * 1 <= 0.000000 + 0]{x2 = 0.0 * x0 + 0.0 * x1 + 1.0 * x2 + 0.0; }
  loc15 -> loc3 [order 1] : [ 1.0 * x0 + 0.0 * x1 + 0.004690461613333069 * x2 + -25.626754994201367 * 1 <= 0.000000 + 0]{x2 = 0.0 * x0 + 0.0 * x1 + 1.0 * x2 + 0.0; }
  loc26 -> loc3 [order 1] : [ 1.0 * x0 + 0.0 * x1 + 4.3638345941383034e-05 * x2 + -8.558005453263958 * 1 <= 0.000000 + 0]{x2 = 0.0 * x0 + 0.0 * x1 + 1.0 * x2 + 0.0; }
  loc37 -> loc5 [order 1] : [ -1.0 * x0 + 0.0 * x1 + -0.007981322807939577 * x2 + 34.00250158216207 * 1 <= 0.000000 + 0]{x2 = 0.0 * x0 + 0.0 * x1 + 1.0 * x2 + 0.0; }
  loc24 -> loc6 [order 2] : [ 1.0 * x0 + 0.0 * x1 + 0.0033737683919804144 * x2 + -15.222760191874794 * 1 <= 0.000000 + 0]{x2 = 0.0 * x0 + 0.0 * x1 + 1.0 * x2 + 0.0; }
  loc4 -> loc5 [order 1] : [ -1.0 * x0 + 0.0 * x1 + 0.008513284706568949 * x2 + -8.055040653945083 * 1 <= 0.000000 + 0]{x2 = 0.0 * x0 + 0.0 * x1 + 1.0 * x2 + 0.0; }
  loc6 -> loc29 [order 18] : [ -1.0 * x0 + 0.0 * x1 + 0.008303191136544342 * x2 + -12.674050860371675 * 1 <= 0.000000 + 0]{x2 = 0.0 * x0 + 0.0 * x1 + 1.0 * x2 + 0.0; }
  loc6 -> loc16 [order 12] : [ -1.0 * x0 + 0.0 * x1 + 0.001303972190562151 * x2 + 5.822824196827431 * 1 <= 0.000000 + 0]{x2 = 0.0 * x0 + 0.0 * x1 + 1.0 * x2 + 0.0; }
  loc6 -> loc7 [order 6] : [ -1.0 * x0 + 9.322214419521627e-15 * x1 + 0.0007340330433825512 * x2 + 8.375236264562027 * 1 <= 0.000000 + 0]{x2 = 0.0 * x0 + 0.0 * x1 + 1.0 * x2 + 0.0; }
  loc8 -> loc20 [order 11] : [ 1.0 * x0 + 0.0 * x1 + -0.035456930932159604 * x2 + 63.475190145397775 * 1 <= 0.000000 + 0]{x2 = 0.0 * x0 + 0.0 * x1 + 1.0 * x2 + 0.0; }
  loc19 -> loc3 [order 3] : [ 1.0 * x0 + 0.0 * x1 + -0.0003742880854435835 * x2 + -8.954541759323723 * 1 <= 0.000000 + 0]{x2 = 0.0 * x0 + 0.0 * x1 + 1.0 * x2 + 0.0; }
  loc12 -> loc1 [order 1] : [ 1.0 * x0 + 0.0 * x1 + -0.041925625491995196 * x2 + 78.95741936467743 * 1 <= 0.000000 + 0]{x2 = 0.0 * x0 + 0.0 * x1 + 1.0 * x2 + 0.0; }
  loc21 -> loc2 [order 2] : [ -1.0 * x0 + 0.0 * x1 + -0.0041607476961556525 * x2 + 23.856964363192976 * 1 <= 0.000000 + 0]{x2 = 0.0 * x0 + 0.0 * x1 + 1.0 * x2 + 0.0; }
  loc23 -> loc2 [order 1] : [ -1.0 * x0 + 0.0 * x1 + -0.02192823590867429 * x2 + 76.84689328498413 * 1 <= 0.000000 + 0]{x2 = 0.0 * x0 + 0.0 * x1 + 1.0 * x2 + 0.0; }
  loc2 -> loc1 [order 1] : [ 1.0 * x0 + 4.14104084370459e-14 * x1 + -0.0015180878794616738 * x2 + -6.108832638579679 * 1 <= 0.000000 + 0]{x2 = 0.0 * x0 + 0.0 * x1 + 1.0 * x2 + 0.0; }
  loc13 -> loc1 [order 1] : [ -1.0 * x0 + 0.0 * x1 + 0.004895312940724413 * x2 + -1.5670216933241397 * 1 <= 0.000000 + 0]{x2 = 0.0 * x0 + 0.0 * x1 + 1.0 * x2 + 0.0; }
  loc1 -> loc2 [order 2] : [ -1.0 * x0 + 6.899556208980658e-14 * x1 + 0.0005335279967858565 * x2 + 8.897662337332136 * 1 <= 0.000000 + 0]{x2 = 0.0 * x0 + 0.0 * x1 + 1.0 * x2 + 0.0; }
  loc1 -> loc9 [order 8] : [ -1.0 * x0 + 0.0 * x1 + 0.0024524758321297856 * x2 + 3.5094395700209255 * 1 <= 0.000000 + 0]{x2 = 0.0 * x0 + 0.0 * x1 + 1.0 * x2 + 0.0; }
  loc1 -> loc25 [order 14] : [ -1.0 * x0 + 0.0 * x1 + 0.01340239988136313 * x2 + -18.481074746693597 * 1 <= 0.000000 + 0]{x2 = 0.0 * x0 + 0.0 * x1 + 1.0 * x2 + 0.0; }
  loc3 -> loc1 [order 1] : [ -1.0 * x0 + 0.0 * x1 + 0.006194374810872679 * x2 + -5.614150713965685 * 1 <= 0.000000 + 0]{x2 = 0.0 * x0 + 0.0 * x1 + 1.0 * x2 + 0.0; }
  loc34 -> loc2 [order 1] : [ -1.0 * x0 + 0.0 * x1 + -0.004722754615463518 * x2 + 25.04876356451336 * 1 <= 0.000000 + 0]{x2 = 0.0 * x0 + 0.0 * x1 + 1.0 * x2 + 0.0; }
  loc2 -> loc8 [order 8] : [ 1.0 * x0 + 0.0 * x1 + -0.0011910798394212322 * x2 + -8.259323577489766 * 1 <= 0.000000 + 0]{x2 = 0.0 * x0 + 0.0 * x1 + 1.0 * x2 + 0.0; }
  loc2 -> loc20 [order 14] : [ 1.0 * x0 + 0.0 * x1 + -0.014663766668078239 * x2 + 20.830649975716142 * 1 <= 0.000000 + 0]{x2 = 0.0 * x0 + 0.0 * x1 + 1.0 * x2 + 0.0; }
  loc24 -> loc2 [order 1] : [ 1.0 * x0 + 0.0 * x1 + 0.002420444454991397 * x2 + -13.283872320605155 * 1 <= 0.000000 + 0]{x2 = 0.0 * x0 + 0.0 * x1 + 1.0 * x2 + 0.0; }
  loc35 -> loc2 [order 1] : [ -1.0 * x0 + 0.0 * x1 + -0.013817728578460742 * x2 + 51.75311521015809 * 1 <= 0.000000 + 0]{x2 = 0.0 * x0 + 0.0 * x1 + 1.0 * x2 + 0.0; }
  loc25 -> loc2 [order 1] : [ -1.0 * x0 + 0.0 * x1 + -0.005232969234294097 * x2 + 27.016609040069703 * 1 <= 0.000000 + 0]{x2 = 0.0 * x0 + 0.0 * x1 + 1.0 * x2 + 0.0; }
  loc2 -> loc7 [order 7] : [ -1.0 * x0 + 2.276876339704819e-13 * x1 + -0.00937667274699846 * x2 + 33.42429243856636 * 1 <= 0.000000 + 0]{x2 = 0.0 * x0 + 0.0 * x1 + 1.0 * x2 + 0.0; }
  loc2 -> loc19 [order 13] : [ 1.0 * x0 + 9.998928431239262e-14 * x1 + -0.004983605070493775 * x2 + 2.5122014608637047 * 1 <= 0.000000 + 0]{x2 = 0.0 * x0 + 0.0 * x1 + 1.0 * x2 + 0.0; }
  loc13 -> loc2 [order 2] : [ 0.0 * x0 + 0.0 * x1 + 3.851905060567147 * x2 + -7770.566595252084 * 1 <= 0.000000 + 0]{x2 = 0.0 * x0 + 0.0 * x1 + 1.0 * x2 + 0.0; }
  loc3 -> loc7 [order 7] : [ 1.0 * x0 + 0.0 * x1 + 0.002659971740094052 * x2 + -13.819030459653218 * 1 <= 0.000000 + 0]{x2 = 0.0 * x0 + 0.0 * x1 + 1.0 * x2 + 0.0; }
  loc3 -> loc27 [order 13] : [ -1.0 * x0 + 0.0 * x1 + 0.012881026541468698 * x2 + -26.16916132259369 * 1 <= 0.000000 + 0]{x2 = 0.0 * x0 + 0.0 * x1 + 1.0 * x2 + 0.0; }
  loc21 -> loc3 [order 3] : [ 1.0 * x0 + 0.0 * x1 + -4.164355661625837e-05 * x2 + -8.41231578823653 * 1 <= 0.000000 + 0]{x2 = 0.0 * x0 + 0.0 * x1 + 1.0 * x2 + 0.0; }
  loc7 -> loc5 [order 4] : [ 1.0 * x0 + -7.690254935082161e-14 * x1 + -0.014688831562219345 * x2 + 23.887468234247542 * 1 <= 0.000000 + 0]{x2 = 0.0 * x0 + 0.0 * x1 + 1.0 * x2 + 0.0; }
  loc9 -> loc5 [order 3] : [ 1.0 * x0 + 0.0 * x1 + 2.019939370557088 * x2 + -4054.854533714733 * 1 <= 0.000000 + 0]{x2 = 0.0 * x0 + 0.0 * x1 + 1.0 * x2 + 0.0; }
  loc11 -> loc5 [order 2] : [ -1.0 * x0 + 0.0 * x1 + -0.02226375312504945 * x2 + 75.98439221129058 * 1 <= 0.000000 + 0]{x2 = 0.0 * x0 + 0.0 * x1 + 1.0 * x2 + 0.0; }
  loc5 -> loc6 [order 6] : [ 1.0 * x0 + 0.0 * x1 + -0.0009842092952084631 * x2 + -7.438667269081777 * 1 <= 0.000000 + 0]{x2 = 0.0 * x0 + 0.0 * x1 + 1.0 * x2 + 0.0; }
  loc5 -> loc16 [order 12] : [ 1.0 * x0 + 0.0 * x1 + -0.024867128450142245 * x2 + 42.883549766594044 * 1 <= 0.000000 + 0]{x2 = 0.0 * x0 + 0.0 * x1 + 1.0 * x2 + 0.0; }
  loc5 -> loc30 [order 18] : [ 1.0 * x0 + 0.0 * x1 + -0.022966929816238688 * x2 + 38.87707668573698 * 1 <= 0.000000 + 0]{x2 = 0.0 * x0 + 0.0 * x1 + 1.0 * x2 + 0.0; }
  loc8 -> loc5 [order 4] : [ 1.0 * x0 + 0.0 * x1 + -0.010250223781191043 * x2 + 13.825397316468143 * 1 <= 0.000000 + 0]{x2 = 0.0 * x0 + 0.0 * x1 + 1.0 * x2 + 0.0; }
  loc14 -> loc5 [order 1] : [ -1.0 * x0 + 0.0 * x1 + -0.07468047483976985 * x2 + 229.52541765301365 * 1 <= 0.000000 + 0]{x2 = 0.0 * x0 + 0.0 * x1 + 1.0 * x2 + 0.0; }
  loc5 -> loc13 [order 11] : [ 1.0 * x0 + 0.0 * x1 + -0.010593891118428875 * x2 + 13.428177035009877 * 1 <= 0.000000 + 0]{x2 = 0.0 * x0 + 0.0 * x1 + 1.0 * x2 + 0.0; }
  loc5 -> loc23 [order 17] : [ -1.0 * x0 + 0.0 * x1 + -0.006877600009965096 * x2 + 31.918686587526622 * 1 <= 0.000000 + 0]{x2 = 0.0 * x0 + 0.0 * x1 + 1.0 * x2 + 0.0; }
  loc22 -> loc6 [order 2] : [ -1.0 * x0 + 0.0 * x1 + 0.009265214325418167 * x2 + -16.633976404134472 * 1 <= 0.000000 + 0]{x2 = 0.0 * x0 + 0.0 * x1 + 1.0 * x2 + 0.0; }
  loc19 -> loc6 [order 4] : [ -1.0 * x0 + 0.0 * x1 + -0.0010323898483073535 * x2 + 14.427707343281915 * 1 <= 0.000000 + 0]{x2 = 0.0 * x0 + 0.0 * x1 + 1.0 * x2 + 0.0; }
  loc6 -> loc14 [order 11] : [ 1.0 * x0 + 0.0 * x1 + 0.07269865119593656 * x2 + -224.27027323897758 * 1 <= 0.000000 + 0]{x2 = 0.0 * x0 + 0.0 * x1 + 1.0 * x2 + 0.0; }
  loc6 -> loc27 [order 17] : [ -1.0 * x0 + 0.0 * x1 + 0.01382943029395847 * x2 + -28.679063337486376 * 1 <= 0.000000 + 0]{x2 = 0.0 * x0 + 0.0 * x1 + 1.0 * x2 + 0.0; }
  loc23 -> loc6 [order 2] : [ -1.0 * x0 + 0.0 * x1 + -0.00303788191864953 * x2 + 20.398700800925084 * 1 <= 0.000000 + 0]{x2 = 0.0 * x0 + 0.0 * x1 + 1.0 * x2 + 0.0; }
  loc7 -> loc6 [order 5] : [ -1.0 * x0 + 0.0 * x1 + -0.0029425001311118443 * x2 + 19.98412187620761 * 1 <= 0.000000 + 0]{x2 = 0.0 * x0 + 0.0 * x1 + 1.0 * x2 + 0.0; }
  loc9 -> loc6 [order 4] : [ 1.0 * x0 + 0.0 * x1 + 0.0017764935686844937 * x2 + -12.004283633454994 * 1 <= 0.000000 + 0]{x2 = 0.0 * x0 + 0.0 * x1 + 1.0 * x2 + 0.0; }
  loc11 -> loc7 [order 3] : [ -1.0 * x0 + 0.0 * x1 + -0.02507818022641773 * x2 + 84.2777321198486 * 1 <= 0.000000 + 0]{x2 = 0.0 * x0 + 0.0 * x1 + 1.0 * x2 + 0.0; }
  loc13 -> loc8 [order 7] : [ -1.0 * x0 + 0.0 * x1 + 0.20048601361455107 * x2 + -395.728855991515 * 1 <= 0.000000 + 0]{x2 = 0.0 * x0 + 0.0 * x1 + 1.0 * x2 + 0.0; }
  loc8 -> loc16 [order 10] : [ 1.0 * x0 + 0.0 * x1 + -0.04540077821578353 * x2 + 87.30601646181007 * 1 <= 0.000000 + 0]{x2 = 0.0 * x0 + 0.0 * x1 + 1.0 * x2 + 0.0; }
  loc8 -> loc34 [order 16] : [ -1.0 * x0 + 0.0 * x1 + 0.008289608083262675 * x2 + -13.960761514383323 * 1 <= 0.000000 + 0]{x2 = 0.0 * x0 + 0.0 * x1 + 1.0 * x2 + 0.0; }
  loc12 -> loc8 [order 2] : [ 1.0 * x0 + 0.0 * x1 + -0.016945000406337785 * x2 + 26.700152448020848 * 1 <= 0.000000 + 0]{x2 = 0.0 * x0 + 0.0 * x1 + 1.0 * x2 + 0.0; }
  loc13 -> loc9 [order 8] : [ -1.0 * x0 + 0.0 * x1 + 0.0008391666839407338 * x2 + 6.757535039051222 * 1 <= 0.000000 + 0]{x2 = 0.0 * x0 + 0.0 * x1 + 1.0 * x2 + 0.0; }
  loc36 -> loc23 [order 1] : [ 1.0 * x0 + 0.0 * x1 + -0.0010961060380068328 * x2 + -8.05797980824718 * 1 <= 0.000000 + 0]{x2 = 0.0 * x0 + 0.0 * x1 + 1.0 * x2 + 0.0; }
  data: x0 input; x1 input; x2_out output; x2 local double; a2 parameter
  data x2 settings: updateMethod=SF_CONTINUOUS_TIME_DATA
